simulink library "thc"  (R2021b)
settings: Solver=VariableStepAuto  StartTime=0.0  StopTime=10.0  RelTol=1e-3
undefined symbols (not defined in the file or in its folder): ATHC_APTCQA_X_C, ATHC_APTCQB_X_C, ATHC_dAy_X_C, ATHC_Qeq_X_kmh, ATHC_VbaseC_X_C, ATHC_VbaseC_Y_W, ATHC_VbaseD_X_C, ATHC_VbaseH_X_C, FALSE, KTHC_ACMaxMinT_sec, KTHC_aDeice_K, KTHC_AGSDefLv_K, KTHC_AGSLv1_K, KTHC_AGSLv2_K, KTHC_AGSLv3_K, KTHC_AGSLv4_K, KTHC_AGSLv5_K, KTHC_AirIntUpdateT_sec, KTHC_APTCOneZoneMax_W, KTHC_APTCQMaxC_W, KTHC_APTCQminC_W, KTHC_APTCQminD_W, KTHC_APTCQminRe1_W, KTHC_APTCQminRe_W, KTHC_APTCQoffT_cnt, KTHC_APTCQonT_cnt, KTHC_APTCRiLeMaxDff_W, KTHC_APTCRiLeMinDff_W, KTHC_BatInTempDef_C, KTHC_bDeice_K, KTHC_CompMaxDeice_rpm, KTHC_CompMinDeice_rpm, KTHC_CompSotxvOp_K, KTHC_CompSotxvOpLow_rpm, KTHC_CompSpdmax_rpm, KTHC_CompSpdmaxBC1_rpm, KTHC_CompSpdmaxBC_rpm, KTHC_CompSpdmid1_rpm, KTHC_CompSpdmid2_rpm, KTHC_CompSpdmid3_rpm, KTHC_CompSpdmid_rpm, KTHC_CompSpdmin_rpm, KTHC_DAPTCQ1_W, KTHC_DAPTCQ2_W, KTHC_DAPTCQ3_W, KTHC_DcChSetTemp_C, KTHC_DehumidityEN_flg, KTHC_DeiceCycTime_K, KTHC_DTambSat1_C, KTHC_DTambSat2_C, KTHC_DTambsat3_C, KTHC_DTambsat4_C, KTHC_DTambSat5_C, KTHC_DTambSat_C, KTHC_DTcabin10_C, KTHC_DTCabin11_C, KTHC_DTcabin12_C, KTHC_DTcabin1_C, KTHC_DTcabin2_C, KTHC_DTcabin3_C ... (+347)
libraries: simulink x80
(part 6 of 8)

== stateflow chart thc/THC/ThermalControl/AC/Chart ==
  state Sync [parallel]
    settings: executionOrder=1
    state WaitForIVI
    state Release
    state Press
      state Wait
      state Over10sec
        en:ACForceOFF=!ACForceOFF;
      (default) -> Wait
      Wait -> Over10sec : [after(100,tick)]
    (default) -> WaitForIVI : {CCU_SyncSts=EEP_CCUSyncSts;ACForceOFF=EEP_ACForceOFF;}
    WaitForIVI -> Sync.Release : [VINP_CANMsgValidIVI2_flg]
    Sync.Release -> Sync.Release [order 2] : [hasChanged(sigSetTempZon2Req_CMD)&&....
        | (sigSetTempZon2Req_CMD) != (sigSetTempZon1Req_CMD)]
        | {CCU_SyncSts=false;}
    Sync.Release -> Sync.Press [order 1] : [FCP_FrEvt_BtnSyncReq]
        | {CCU_SyncSts=!CCU_SyncSts;}
    Sync.Press -> Sync.Release [order 1] : [!FCP_FrEvt_BtnSyncReq]
    Sync.Press -> Sync.Press [order 2] : [hasChanged(sigSetTempZon2Req_CMD)&&....
        | (sigSetTempZon2Req_CMD) != (sigSetTempZon1Req_CMD)]
        | {CCU_SyncSts=false;}
  state Recycle [parallel]
    settings: executionOrder=13
    state Manual
      state Outter
        en:sigRecircSt=false;
        state ACOFF
          en:FD_RecyAuto_Cmd=0;
        state ACON
          en:FD_RecyAuto_Cmd=4;
        (default) -> (junction 1044)
        (junction 1044) -> ACOFF [order 1] : [!CCU_ACLampSts&&....
            | (CabinMode==11&&....
            | ACSubMode==1)]
        (junction 1044) -> ACON [order 2]
        ACON -> ACOFF : [!CCU_ACLampSts&&....
            | (CabinMode==11&&ACSubMode==1)]
        ACOFF -> ACON : [CCU_ACLampSts||....
            | (CabinMode!=11||ACSubMode!=1)]
      state Inner
        en:sigRecircSt=true;
        FD_RecyAuto_Cmd=0;
      (default) -> (junction 920)
      (junction 920) -> (junction 922) [order 1] : [EEP_sigRecircSt]
      (junction 920) -> Outter [order 2]
      (junction 922) -> Inner
      Inner -> Outter [order 2] : eDefogRecycle
      Outter -> Inner : eRecycleBtn
      Inner -> Outter [order 1] : eRecycleBtn
      (junction 839) -> Outter [order 1] : [sigRecircSt]
      (junction 839) -> Inner [order 2]
    state Auto
      state SetLowT
        en:sigRecircSt=false;FD_RecyAuto_Cmd=4;
      state Normal
        state AutoInner
          en:
          sigRecircSt=true;
          note: 2 min
          state Refresh
            en:
            FD_RecyAuto_Cmd=4;
          state Hold
            en:
            FD_RecyAuto_Cmd=0;
          (default) -> Hold
          Refresh -> Hold : [after(KTHC_RecyChange_min*600,tick)]
          Hold -> Refresh : [KTHC_RefreshEN_flg&&...
              | after(KTHC_RecyHold_min*600,tick)]
        note: 30 min
        state AutoOutter
          en:sigRecircSt=false;
          state Dehumidity
            en:FD_RecyAuto_Cmd=KTHC_RecyOutterD_enum;
          state Normal
            state LV5
              en:FD_RecyAuto_Cmd=4;
            state LV4
              en:FD_RecyAuto_Cmd=3;
            state LV3
              en:FD_RecyAuto_Cmd=2;
            state LV2
              en:FD_RecyAuto_Cmd=1;
            (junction 713) -> LV5 [order 1] : [Tamb>KTHC_T4Mmaxamb_C]
            (junction 713) -> (junction 719) [order 2]
            LV5 -> LV4 : [Tamb<KTHC_T5Mminamb_C]
            LV4 -> LV5 [order 1] : [Tamb>KTHC_T4Mmaxamb_C]
            (junction 719) -> LV4 [order 1] : [Tamb>KTHC_T3Mmaxamb_C]
            (junction 719) -> (junction 725) [order 2]
            LV4 -> LV3 [order 2] : [Tamb<KTHC_T4Mminamb_C]
            LV3 -> LV4 [order 1] : [Tamb>KTHC_T3Mmaxamb_C]
            (junction 725) -> LV3 [order 1] : [Tamb>KTHC_T2Mmaxamb_C]
            (junction 725) -> (junction 730) [order 2]
            LV3 -> LV2 [order 2] : [Tamb<KTHC_T3Mminamb_C]
            LV2 -> LV3 : [Tamb>KTHC_T2Mmaxamb_C]
            (junction 730) -> LV2
          (default) -> (junction 1030)
          (junction 1030) -> Dehumidity [order 1] : [CabinMode<7]
          (junction 1030) -> (junction 1034) [order 2]
          Dehumidity -> (junction 1034) : [CabinMode>=7]
          (junction 1034) -> (junction 713)
          Recycle.Auto.Normal.AutoOutter.Normal -> Dehumidity : [CabinMode<7]
        (default) -> (junction 752)
        (junction 752) -> AutoInner [commented out] : [CabinMode==3||....
            | CabinMode==6||....
            | (CabinMode==11&&....
            | ACSubMode==1)]
        (junction 752) -> (junction 754)
        AutoInner -> (junction 754) : [CabinMode!=3&&....
            | CabinMode!=6&&....
            | (CabinMode!=11||....
            | ACSubMode!=1)]
        (junction 754) -> AutoOutter
        AutoOutter -> AutoInner : [CabinMode==3||CabinMode==6||....
            | (CabinMode==11&&ACSubMode==1)]
      (default) -> (junction 1010)
      (junction 1010) -> (junction 1014) [order 1]
      (junction 1014) -> SetLowT : [CabinMode==3&&(ACSubMode==2||ACSubMode==6||ACSubMode==7)....
          | &&SetTempZon1St_CMD==170&&Tamb<KTHC_Trecymin_C]
      SetLowT -> Recycle.Auto.Normal : [CabinMode!=3||(ACSubMode!=2&&ACSubMode!=6&&ACSubMode!=7)||....
          | SetTempZon1St_CMD>170||Tamb>=KTHC_Trecymin_C]
      (junction 1010) -> Recycle.Auto.Normal [order 2]
      Recycle.Auto.Normal -> (junction 1014)
    (default) -> (junction 914)
    (junction 914) -> Recycle.Manual [order 1] : [EEP_ACModeMem!=2||!EEP_RecAutoFlg]
        | {RecAutoFlg=EEP_RecAutoFlg;}
    (junction 914) -> (junction 917) [order 2]
    Recycle.Auto -> (junction 839) [order 3] : eRecycleBtn
    Recycle.Auto -> Outter [order 2] : [!CCU_AutoLampSts&&!RecAutoFlg&&!sigRecircSt]
    Recycle.Auto -> Outter [order 1] : eDefogRecycle
    Recycle.Auto -> Inner [order 4] : [!CCU_AutoLampSts&&!RecAutoFlg]
    Recycle.Manual -> Recycle.Auto [order 2] : eACMaxRec
    Recycle.Manual -> Recycle.Auto [order 1] : [CCU_AutoLampSts&&RecAutoFlg]
    (junction 917) -> Recycle.Auto
  state RecycleSW [parallel]
    settings: executionOrder=14
    state Release
    state Press
      en:Recycle.eRecycleBtn;
      RecAutoFlg=false;
    (default) -> RecycleSW.Release
    RecycleSW.Release -> RecycleSW.Press : [sigRecircReq]
    RecycleSW.Press -> RecycleSW.Release : [!sigRecircReq]
  state PETMODE [parallel]
    settings: executionOrder=16
    state OFF
      en:PET=false;
    state ON
      en:PET=true;
    (default) -> PETMODE.OFF
    PETMODE.OFF -> PETMODE.ON : [(PwrSta>0&&PwrSta<=3&&(OFF_AC_MODE==1||OFF_AC_MODE==2||VINP_RemoteAutoReq_flg))||(ForceAuto&&PwrSta>3)]
    PETMODE.ON -> PETMODE.OFF : [(PwrSta==0||PwrSta>3||(OFF_AC_MODE!=1&&OFF_AC_MODE!=2&&!VINP_RemoteAutoReq_flg))&&(!ForceAuto||PwrSta<=3)]
  state ACBtn [parallel]
    settings: executionOrder=2
    state Initial
    state Release
    state Press
      en:AC.ACMode.eACBtn;
      WaterFill.eACBtn;
    (default) -> ACBtn.Initial
    ACBtn.Initial -> (junction 899) [order 2]
    (junction 899) -> ACBtn.Press
    ACBtn.Initial -> ACBtn.Release [order 1] : [EEP_ACModeMem!=1]
    ACBtn.Press -> ACBtn.Release : [!FCP_FrEvt_BtnACReq]
    ACBtn.Release -> ACBtn.Press : [FCP_FrEvt_BtnACReq]
  state ACAutoBtn [parallel]
    settings: executionOrder=3
    state Initial
    state Release
    state Press
      en:
      WaterFill.eACAutoBtn;
      RecAutoFlg=true;
    (default) -> ACAutoBtn.Initial
    ACAutoBtn.Initial -> (junction 904) [order 2] : {AC.ACMode.eACAutoBtn;}
    (junction 904) -> ACAutoBtn.Release
    ACAutoBtn.Initial -> ACAutoBtn.Release [order 1] : [EEP_ACModeMem!=2]
    ACAutoBtn.Release -> (junction 700) : [FCP_FrEvt_BtnAutoReq]
    (junction 700) -> ACAutoBtn.Press [order 1] : [CCU_AutoLampSts]{AC.ACMode.eAutoexit;}
    (junction 700) -> (junction 702) [order 2]
    (junction 702) -> ACAutoBtn.Press : {AC.ACMode.eACAutoBtn;}
    ACAutoBtn.Press -> ACAutoBtn.Release : [!FCP_FrEvt_BtnAutoReq]
  state ACMaxBtn [parallel]
    settings: executionOrder=4
    state Release
    state Press
      en:AC.ACMode.eACMaxBtn;
    (default) -> ACMaxBtn.Release
    ACMaxBtn.Release -> ACMaxBtn.Press : [FCP_FrEvt_BtnACMaxReq]
    ACMaxBtn.Press -> ACMaxBtn.Release : [!FCP_FrEvt_BtnACMaxReq]
  state FaceBtn [parallel]
    settings: executionOrder=5
    state Press
      en:AC.ACMode.eAutoexit;
    state Release
    (default) -> FaceBtn.Release : {Face=EEP_Face;}
    FaceBtn.Press -> FaceBtn.Release : [!sigFaceReq]
    FaceBtn.Release -> (junction 183) : [sigFaceReq]{fdefog=false;}
    (junction 183) -> FaceBtn.Press [order 1] : [Face&&!Foot&&!Frost]
    (junction 183) -> (junction 185) [order 2]
    (junction 185) -> FaceBtn.Press : {Face=!Face;}
  state FootBtn [parallel]
    settings: executionOrder=6
    state Release
    state Press
      en:AC.ACMode.eAutoexit;
    (default) -> FootBtn.Release : {Foot=EEP_Foot;}
    FootBtn.Press -> FootBtn.Release : [!sigFootReq]
    FootBtn.Release -> (junction 189) : [sigFootReq]{fdefog=false;}
    (junction 189) -> FootBtn.Press [order 1] : [!Face&&Foot&&!Frost]
    (junction 189) -> (junction 197) [order 2]
    (junction 197) -> FootBtn.Press : {Foot=!Foot;}
  state Frost [parallel]
    settings: executionOrder=7
    state Press
      en:AC.ACMode.eAutoexit;
      ACModeMem=1;
    state Release
    (default) -> Frost.Release : {Frost=EEP_Frost;FaceM=EEP_FaceM;FootM=EEP_FootM;fdefog=EEP_fdefog;}
    Frost.Press -> Frost.Release : [!sigFrostReq]
    Frost.Release -> (junction 206) : [sigFrostReq]
    (junction 206) -> Frost.Press [order 1] : [!Frost]{Frost=true;FaceM=Face;FootM=Foot;....
        | Face=false;Foot=false;fdefog=true;Recycle.eDefogRecycle;RecAutoFlg=false;}
    (junction 206) -> (junction 200) [order 2]
    (junction 200) -> Frost.Press [order 1] : [!Face&&!Foot]{Frost=false;Face=FaceM;Foot=FootM;fdefog=false;}
    (junction 200) -> (junction 769) [order 2]
    (junction 769) -> Frost.Press : {Frost=false;fdefog=false;}
  state AC [parallel]
    settings: executionOrder=15
    state ACMode
      state ON
        state Max
          en:
          CCU_ACLampSts=true;
          CCU_AutoLampSts=false;
          CCU_ACMaxLampSts=true;
          sigAirIntenZon1St=9;
          CCU_SyncSts=true;
          Recycle.eACMaxRec;
          RecAutoFlg=true;
          state WaitMinT
          state WaitFinish
          (default) -> WaitMinT
          WaitMinT -> WaitFinish : [after(KTHC_ACMaxMinT_sec*10,tick)]
        state Manual
          en:
          CCU_ACLampSts=true;CCU_AutoLampSts=false;
          CCU_ACMaxLampSts=false;ACModeMem=1;
          RecAutoFlg=false;
          ACModeMem = 1;
          state Normal
            en:
            sigAirIntenZon1St=AirIntenZone1M;
            du:
            sigAirIntenZon1St=AirIntenZone1M;
          state DeFog
            en:
            sigAirIntenZon1St=9;
            ex:
            fdefog=false;
          (default) -> (junction 779)
          (junction 779) -> DeFog [order 2]
          (junction 779) -> AC.ACMode.ON.Manual.Normal [order 1] : [!fdefog]
          DeFog -> AC.ACMode.ON.Manual.Normal : [!fdefog]
          AC.ACMode.ON.Manual.Normal -> DeFog : [fdefog]
        state Auto
          en:
          CCU_ACLampSts=true;
          CCU_AutoLampSts=true;
          CCU_ACMaxLampSts=false;
          ACModeMem=2;
        WaitFinish -> (junction 851) : [MaxFinish||....
            | !CCU_SyncSts]
        Max -> AC.ACMode.ON.Manual [order 2] : eACMaxexit
        AC.ACMode.ON.Manual -> Max : eACMaxBtn
        Max -> (junction 850) [order 1] : eACMaxBtn
        AC.ACMode.ON.Auto -> Max [order 1] : eACMaxBtn
        (junction 850) -> (junction 851)
        (junction 851) -> (junction 49)
        (junction 49) -> AC.ACMode.ON.Manual [order 2]
        (junction 49) -> AC.ACMode.ON.Auto [order 1] : [ACModeMem==2]
        AC.ACMode.ON.Auto -> AC.ACMode.ON.Manual [order 2] : eAutoexit
        AC.ACMode.ON -> AC.ACMode.ON.Auto [order 1] : eACAutoBtn
        (default) -> (junction 943)
        (junction 943) -> AC.ACMode.ON.Manual [order 2]
        (junction 943) -> AC.ACMode.ON.Auto [order 1] : [ACModeMem == 2]
      state OFF
        en:
        CCU_ACLampSts=false;
        CCU_AutoLampSts=false;
        CCU_ACMaxLampSts=false;
        ACModeMem=0;
        sigAirIntenZon1St=AirIntenZone1M;
        du:
        sigAirIntenZon1St=AirIntenZone1M;
      (default) -> AC.ACMode.OFF
      AC.ACMode.OFF -> (junction 669) [order 4] : eACMaxBtn{ACModeMem=1;}
      (junction 669) -> Max [order 1] : [AirIntenZone1M!=1]
      (junction 669) -> (junction 671) [order 2]
      (junction 671) -> Max : {AirIntenZone1M=2;}
      AC.ACMode.ON -> AC.ACMode.OFF [order 1] : eACBtn
      AC.ACMode.OFF -> (junction 832) [order 2] : eACBtn
      (junction 832) -> (junction 833)
      AC.ACMode.OFF -> (junction 833) [order 1] : [fdefog]
      (junction 833) -> (junction 674)
      (junction 674) -> AC.ACMode.ON.Manual [order 1] : [AirIntenZone1M!=1]
      (junction 674) -> (junction 677) [order 2]
      (junction 677) -> AC.ACMode.ON.Manual : {AirIntenZone1M=2;}
      AC.ACMode.ON -> AC.ACMode.OFF [order 2] : [sigAirIntenZon1Req==1]
      (junction 683) -> AC.ACMode.ON.Auto [order 1] : [AirIntenZone1M!=1]
      AC.ACMode.OFF -> (junction 683) [order 3] : eACAutoBtn
      (junction 683) -> (junction 680) [order 2]
      (junction 680) -> AC.ACMode.ON.Auto : {AirIntenZone1M=2;}
      (junction 948) -> AC.ACMode.OFF [order 1] : [ACModeMem == 0]
      (junction 948) -> AC.ACMode.ON [order 2]
      (junction 947) -> (junction 948)
    state PET
      en:
      CCU_ACLampSts=true;
      CCU_AutoLampSts=true;
      CCU_ACMaxLampSts=false;
    (default) -> ACMode
    ACMode -> PET : [PET]
    PET -> (junction 947) : [!PET]
  state AutoWindDir [parallel]
    settings: executionOrder=12
    state Manmual
    state Standby
    (default) -> (junction 560)
    (junction 560) -> Manmual [order 1] : [!CCU_AutoLampSts]
    (junction 560) -> (junction 871) [order 2]
    Standby -> (junction 871) [order 3] : [hasChanged(VTHC_FootCold_flg)]
    (junction 871) -> (junction 578)
    Manmual -> (junction 578) : [CCU_AutoLampSts]
    Standby -> (junction 578) [order 1] : [after(KTHC_WindDirUpdateT_min*600,tick)||hasChanged(SetTempZon1St_CMD)]
    (junction 578) -> (junction 562)
    (junction 562) -> (junction 568) [order 1] : [Tamb<20]
    (junction 568) -> Standby [order 1] : [sigSetTempZon1St<Tincar||VTHC_FootCold_flg]....
        | {Face=KTHC_WDZ2Face_flg;Foot=KTHC_WDZ2Foot_flg;Frost=KTHC_WDZ2Frost_flg;}
    (junction 562) -> (junction 573) [order 2]
    (junction 568) -> (junction 570) [order 2]
    (junction 570) -> Standby : {Face=KTHC_WDZ1Face_flg;Foot=KTHC_WDZ1Foot_flg;Frost=KTHC_WDZ1Frost_flg;}
    (junction 575) -> Standby [order 1] : [Tincar-Tamb>KTHC_Tmidlevel_C]....
        | {Face=KTHC_WDZ5Face_flg;Foot=KTHC_WDZ5Foot_flg;Frost=KTHC_WDZ5Frost_flg;}
    (junction 573) -> (junction 575) [order 1] : [Tamb<25]
    (junction 573) -> (junction 581) [order 2]
    (junction 575) -> (junction 605) [order 2]
    (junction 605) -> Standby [order 1] : [sigSetTempZon1St<Tincar||VTHC_FootCold_flg]....
        | {Face=KTHC_WDZ3Face_flg;Foot=KTHC_WDZ3Foot_flg;Frost=KTHC_WDZ3Frost_flg;}
    (junction 605) -> (junction 608) [order 2]
    (junction 608) -> Standby : {Face=KTHC_WDZ4Face_flg;Foot=KTHC_WDZ4Foot_flg;Frost=KTHC_WDZ4Frost_flg;}
    (junction 624) -> Standby [order 1] : [sigSetTempZon1St<Tincar]....
        | {Face=KTHC_WDZ9Face_flg;Foot=KTHC_WDZ9Foot_flg;Frost=KTHC_WDZ9Frost_flg;}
    (junction 581) -> (junction 624) [order 1] : [Tincar-Tamb>KTHC_Thilevel2_C]
    (junction 581) -> (junction 583) [order 2]
    (junction 624) -> (junction 625) [order 2]
    (junction 625) -> Standby : {Face=KTHC_WDZ8Face_flg;Foot=KTHC_WDZ8Foot_flg;Frost=KTHC_WDZ8Frost_flg;}
    (junction 1051) -> (junction 625) [order 2]
    (junction 583) -> (junction 1051) [order 1] : [Tincar-Tamb>KTHC_Thilevel1_C]
    (junction 1051) -> Standby [order 1] : [sigSetTempZon1St<Tincar]....
        | {Face=KTHC_WDZ10Face_flg;Foot=KTHC_WDZ10Foot_flg;Frost=KTHC_WDZ10Frost_flg;}
    (junction 583) -> (junction 586) [order 2]
    (junction 586) -> Standby [order 1] : [sigSetTempZon1St>=Tincar]....
        | {Face=KTHC_WDZ7Face_flg;Foot=KTHC_WDZ7Foot_flg;Frost=KTHC_WDZ7Frost_flg;}
    (junction 586) -> (junction 589) [order 2]
    (junction 589) -> Standby : {Face=KTHC_WDZ6Face_flg;Foot=KTHC_WDZ6Foot_flg;Frost=KTHC_WDZ6Frost_flg;}
    Standby -> Manmual [order 2] : [!CCU_AutoLampSts]
  state WindDir [parallel]
    settings: executionOrder=8
    state Face
      en:sigWindDirZon1St=0;
    state Bilevel
      en:sigWindDirZon1St=1;
    state Foot
      en:sigWindDirZon1St=2;
    state FootandScreen
      en:sigWindDirZon1St=3;
    state Defog
      en:sigWindDirZon1St=4;
    state FaceandScreen
      en:sigWindDirZon1St=5;
    state AllOpen
      en:sigWindDirZon1St=6;
    state AllClose
      en:sigWindDirZon1St=7;
    (default) -> (junction 457)
    WindDir -> (junction 457) : [hasChanged(Face)||....
        | hasChanged(Foot)||....
        | hasChanged(Frost)]
    (junction 457) -> Face [order 1] : [Face&&!Foot&&!Frost]
    (junction 457) -> (junction 464) [order 2]
    (junction 464) -> Bilevel [order 1] : [Face&&Foot&&!Frost]
    (junction 464) -> (junction 467) [order 2]
    (junction 467) -> Foot [order 1] : [!Face&&Foot&&!Frost]
    (junction 467) -> (junction 472) [order 2]
    (junction 472) -> FootandScreen [order 1] : [!Face&&Foot&&Frost]
    (junction 472) -> (junction 476) [order 2]
    (junction 476) -> Defog [order 1] : [!Face&&!Foot&&Frost]
    (junction 476) -> (junction 480) [order 2]
    (junction 480) -> FaceandScreen [order 1] : [Face&&!Foot&&Frost]
    (junction 480) -> (junction 484) [order 2]
    (junction 484) -> AllOpen [order 1] : [Face&&Foot&&Frost]
    (junction 484) -> AllClose [order 2]
  state Manual [parallel]
    settings: executionOrder=10
    state Updated
      en:AC.ACMode.eAutoexit;
      CCU_AutoLampSts=false;
    state Auto
      state WaitForUpdate
      (default) -> (junction 953) : {FAutoFirst=true;}
      WaitForUpdate -> (junction 953) [order 2] : [after(2,tick)&&FAutoFirst]{FAutoFirst=false;}
      (junction 953) -> (junction 954)
      WaitForUpdate -> (junction 954) [order 3] : [FD_Blower_Cmd>AirIntHB||FD_Blower_Cmd<AirIntLB]
      (junction 954) -> (junction 955)
      WaitForUpdate -> (junction 955) [order 1] : [after(KTHC_AirIntUpdateT_sec*10,tick)]
      (junction 955) -> (junction 956)
      (junction 956) -> WaitForUpdate [order 1] : [FD_Blower_Cmd>=94]{sigAirIntenZon1St=9;AirIntLB=87.5;AirIntHB=100;}
      (junction 956) -> (junction 957) [order 2]
      (junction 957) -> WaitForUpdate [order 1] : [FD_Blower_Cmd>=82]{sigAirIntenZon1St=8;AirIntLB=75;AirIntHB=100;}
      (junction 957) -> (junction 958) [order 2]
      (junction 958) -> WaitForUpdate [order 1] : [FD_Blower_Cmd>=69]{sigAirIntenZon1St=7;AirIntLB=62.5;AirIntHB=87.5;}
      (junction 958) -> (junction 959) [order 2]
      (junction 959) -> WaitForUpdate [order 1] : [FD_Blower_Cmd>=56]{sigAirIntenZon1St=6;AirIntLB=50;AirIntHB=75;}
      (junction 959) -> (junction 960) [order 2]
      (junction 960) -> WaitForUpdate [order 1] : [FD_Blower_Cmd>=44]{sigAirIntenZon1St=5;AirIntLB=37.5;AirIntHB=62.5;}
      (junction 960) -> (junction 961) [order 2]
      (junction 961) -> WaitForUpdate [order 1] : [FD_Blower_Cmd>=32]{sigAirIntenZon1St=4;AirIntLB=25;AirIntHB=50;}
      (junction 961) -> (junction 962) [order 2]
      (junction 962) -> WaitForUpdate [order 1] : [FD_Blower_Cmd>=19]{sigAirIntenZon1St=3;AirIntLB=12.5;AirIntHB=37.5;}
      (junction 962) -> (junction 963) [order 2]
      (junction 963) -> WaitForUpdate : {sigAirIntenZon1St=2;;AirIntLB=0;AirIntHB=25;}
    (default) -> (junction 117) : {AirIntenZone1M=EEP_AirIntenZone1M;}
    (junction 117) -> Updated [order 2]
    (junction 117) -> Manual.Auto [order 1] : [CCU_AutoLampSts]
    Updated -> Manual.Auto : [CCU_AutoLampSts]
    Manual.Auto -> Updated : [!CCU_AutoLampSts]
    (junction 817) -> Updated [order 1] : [CCU_ACMaxLampSts]....
        | {AC.ACMode.eACMaxexit;}
    Manual -> (junction 817) : [hasChanged(sigAirIntenZon1Req)&&....
        | sigAirIntenZon1Req>0&&sigAirIntenZon1Req<10]....
        | {AirIntenZone1M=sigAirIntenZon1Req;fdefog=false;}
    (junction 817) -> (junction 819) [order 2]
    (junction 819) -> Updated
  state WaterFill [parallel]
    settings: executionOrder=9
    state Count1
    state OFF
      en:WaterFillReq=0;
      WFCnt=0;
    state Count
      en:WFCnt=WFCnt+1;
    state WaterFill2
      en:WaterFillReq=2;
    state WaterFill1
      en:WaterFillReq=1;
    (default) -> WaterFill.OFF
    WaterFill.OFF -> Count1 [order 2] : [FCP_FrEvt_BtnACReq]
    Count1 -> WaterFill.OFF [order 1] : [!FCP_FrEvt_BtnACReq]
    WaterFill.OFF -> Count [order 1] : eACAutoBtn....
        | [SetTempZon1St_CMD == 220 &&...
        |  SetTempZon2St_CMD == 310]
    Count -> WaterFill.OFF [order 3] : [SetTempZon1St_CMD != 220 ||...
        |  SetTempZon2St_CMD !=310 ||...
        | after(20,tick)]
    WaterFill1 -> WaterFill.OFF [order 1] : eACBtn
    (junction 1005) -> WaterFill.OFF : eACAutoBtn
    (junction 1002) -> WaterFill.OFF [order 1] : [after(36000,tick)||....
        | PwrSta==0||....
        | PwrSta==5]
    Count1 -> WaterFill2 [order 2] : [after(50,tick)]
    Count -> Count [order 2] : eACAutoBtn
    Count -> WaterFill1 [order 1] : [WFCnt>=3]
    (junction 1002) -> (junction 1005) [order 2]
    WaterFill2 -> (junction 1002)
    WaterFill1 -> (junction 1002) [order 2]
  state TFootUpdate [parallel]
    settings: executionOrder=11
    state Low
      en:
      VTHC_FootCold_flg=true;
    state High
      en:
      VTHC_FootCold_flg=false;
    (default) -> (junction 864)
    (junction 864) -> Low [order 1] : [T_Foot_min<KTHC_FootColdT_C]
    (junction 864) -> High [order 2]
    High -> Low : [T_Foot_min<KTHC_FootColdT_C]
    Low -> High : [T_Foot_min>KTHC_FootColdT_C+KTHC_FootColdTdelta_C]
  data: FCP_FrEvt_BtnACMaxReq input; FCP_FrEvt_BtnACReq input; FCP_FrEvt_BtnAutoReq input; FCP_FrEvt_BtnSyncReq input; FD_Blower_Cmd input; Tamb input; Tincar input; sigAirIntenZon1Req input; sigRecircReq input; CCU_ACLampSts output boolean; CCU_ACMaxLampSts output boolean; CCU_SyncSts output; sigAirIntenZon1St output; sigWindDirZon1St output; CCU_AutoLampSts output boolean; sigRecircSt output =0; sigFaceReq input; sigFootReq input; sigFrostReq input; sigSetTempZon1St input; SetTempZon1St_CMD input; sigSetTempZon2St input; SetTempZon2St_CMD input; PwrSta input; sigSetTempZon1Req input; sigSetTempZon2Req_CMD input; sigSetTempZon1Req_CMD input; sigSetTempZon2Req input; WaterFillReq output uint8; WFCnt local uint8; Frost output boolean; ACForceOFF output; KTHC_WindDirUpdateT_min input; KTHC_AirIntUpdateT_sec input; OFF_AC_MODE input; PET output boolean; FD_RecyAuto_Cmd output; KTHC_T2Mmaxamb_C input; KTHC_T3Mmaxamb_C input; KTHC_T4Mmaxamb_C input; KTHC_T3Mminamb_C input; KTHC_T4Mminamb_C input; KTHC_T5Mminamb_C input; KTHC_RecyHold_min input; KTHC_RecyChange_min input; KTHC_Tmidlevel_C input; KTHC_Thilevel1_C input; KTHC_Thilevel2_C input; CabinMode input; KTHC_WDZ1Face_flg input boolean; KTHC_WDZ1Foot_flg input boolean; KTHC_WDZ1Frost_flg input boolean; KTHC_WDZ2Face_flg input boolean; KTHC_WDZ2Foot_flg input boolean; KTHC_WDZ2Frost_flg input boolean; KTHC_WDZ3Face_flg input boolean; KTHC_WDZ3Foot_flg input boolean; KTHC_WDZ3Frost_flg input boolean; KTHC_WDZ4Face_flg input boolean; KTHC_WDZ4Foot_flg input boolean; KTHC_WDZ4Frost_flg input boolean; KTHC_WDZ5Face_flg input boolean; KTHC_WDZ5Foot_flg input boolean; KTHC_WDZ5Frost_flg input boolean; KTHC_WDZ6Face_flg input boolean; KTHC_WDZ6Foot_flg input boolean; KTHC_WDZ6Frost_flg input boolean; KTHC_WDZ7Face_flg input boolean; KTHC_WDZ7Foot_flg input boolean; KTHC_WDZ7Frost_flg input boolean; KTHC_WDZ8Face_flg input boolean; KTHC_WDZ8Foot_flg input boolean; KTHC_WDZ8Frost_flg input boolean; KTHC_WDZ9Face_flg input boolean; KTHC_WDZ9Foot_flg input boolean; KTHC_WDZ9Frost_flg input boolean; KTHC_WDZ10Face_flg input; KTHC_WDZ10Foot_flg input; KTHC_WDZ10Frost_flg input; ForceAuto input; KTHC_RefreshEN_flg input boolean; MaxFinish input; T_Foot_min input; KTHC_FootColdT_C input; KTHC_FootColdTdelta_C input; VTHC_FootCold_flg local boolean; KTHC_ACMaxMinT_sec input; FAutoFirst local boolean; ACModeMem output; EEP_ACModeMem input; EEP_Face input; EEP_Foot input; EEP_Frost input; EEP_FaceM input; EEP_FootM input; FaceM output boolean; FootM output boolean; Face output boolean; Foot output boolean; EEP_CCUSyncSts input; EEP_ACForceOFF input; EEP_sigRecircSt input; EEP_RecAutoFlg input; EEP_AirIntenZone1M input; EEP_fdefog input; fdefog output boolean; RecAutoFlg output boolean; AirIntenZone1M output; VINP_CANMsgValidIVI2_flg input; VINP_RemoteAutoReq_flg input; AirIntHB local double; AirIntLB local double; KTHC_Trecymin_C input; ACSubMode input; KTHC_RecyOutterD_enum input
  events: eRecycleBtn local FUNCTION_CALL_EVENT; eDefogRecycle local FUNCTION_CALL_EVENT; eACMaxRec local FUNCTION_CALL_EVENT; eACBtn local FUNCTION_CALL_EVENT; eACMaxBtn local FUNCTION_CALL_EVENT; eACAutoBtn local FUNCTION_CALL_EVENT; eAutoexit local FUNCTION_CALL_EVENT; eACMaxexit local FUNCTION_CALL_EVENT; eACAutoBtn local FUNCTION_CALL_EVENT; eACBtn local FUNCTION_CALL_EVENT

== stateflow chart thc/THC/ThermalControl/THCM_Conctrl/Chart2 ==
  state FactorSolar1
    en:FactorSolar=0.88;Blowersolar=1000;
    state Low
    state Mid
    (default) -> FactorSolar1.Mid
    FactorSolar1.Mid -> FactorSolar1.Low : [Solar<950]
    FactorSolar1.Low -> FactorSolar1.Mid [order 1] : [Solar>=950]
  state FactorSolar2
    en:FactorSolar=0.90;Blowersolar=860;
    state Low
    state Mid
    state High
    (default) -> FactorSolar2.Mid
    FactorSolar2.Mid -> FactorSolar2.High [order 2] : [Solar>1000]
    FactorSolar2.Mid -> FactorSolar2.Low [order 1] : [Solar<800]
    FactorSolar2.Low -> FactorSolar2.Mid [order 1] : [Solar>=800]
    FactorSolar2.High -> FactorSolar2.Mid [order 2] : [Solar<=1000]
  state FactorSolar3
    en:FactorSolar=0.92;Blowersolar=715;
    state Low
    state Mid
    state High
    (default) -> FactorSolar3.Mid
    FactorSolar3.Mid -> FactorSolar3.High [order 2] : [Solar>850]
    FactorSolar3.Mid -> FactorSolar3.Low [order 1] : [Solar<650]
    FactorSolar3.Low -> FactorSolar3.Mid [order 1] : [Solar>=650]
    FactorSolar3.High -> FactorSolar3.Mid [order 1] : [Solar<=850]
  state FactorSolar4
    en:FactorSolar=0.94;Blowersolar=570;
    state Low
    state Mid
    state High
    (default) -> FactorSolar4.Mid
    FactorSolar4.Mid -> FactorSolar4.High [order 2] : [Solar>700]
    FactorSolar4.Mid -> FactorSolar4.Low [order 1] : [Solar<500]
    FactorSolar4.Low -> FactorSolar4.Mid [order 1] : [Solar>=500]
    FactorSolar4.High -> FactorSolar4.Mid [order 1] : [Solar<=700]
  state FactorSolar5
    en:FactorSolar=0.96;Blowersolar=430;
    state Low
    state Mid
    state High
    (default) -> FactorSolar5.Mid
    FactorSolar5.Mid -> FactorSolar5.High [order 2] : [Solar>550]
    FactorSolar5.Mid -> FactorSolar5.Low [order 1] : [Solar<350]
    FactorSolar5.Low -> FactorSolar5.Mid [order 1] : [Solar>=350]
    FactorSolar5.High -> FactorSolar5.Mid [order 1] : [Solar<=550]
  state FactorSolar6
    en:FactorSolar=0.98;Blowersolar=285;
    state Low
    state Mid
    state High
    (default) -> FactorSolar6.Mid
    FactorSolar6.Mid -> FactorSolar6.High [order 2] : [Solar>400]
    FactorSolar6.Mid -> FactorSolar6.Low [order 1] : [Solar<200]
    FactorSolar6.Low -> FactorSolar6.Mid : [Solar>=200]
    FactorSolar6.High -> FactorSolar6.Mid [order 1] : [Solar<=400]
  state FactorSolar7
    en:FactorSolar=1;Blowersolar=100;
    state Mid
    state High
    (default) -> FactorSolar7.Mid
    FactorSolar7.Mid -> FactorSolar7.High : [Solar>250]
    FactorSolar7.High -> FactorSolar7.Mid [order 1] : [Solar<=250]
  (default) -> (junction 9)
  (junction 9) -> FactorSolar1 [order 1] : [Solar>950]
  (junction 9) -> (junction 11) [order 2]
  FactorSolar1.Low -> FactorSolar2 [order 2] : [after(KTHC_SolarDebounceT_sec*10,tick)]
  FactorSolar2.High -> FactorSolar1 [order 1] : [after(KTHC_SolarDebounceT_sec*10,tick)]
  (junction 11) -> FactorSolar2 [order 1] : [Solar>800]
  (junction 11) -> (junction 14) [order 2]
  FactorSolar2.Low -> FactorSolar3 [order 2] : [after(KTHC_SolarDebounceT_sec*10,tick)]
  FactorSolar3.High -> FactorSolar2 [order 2] : [after(KTHC_SolarDebounceT_sec*10,tick)]
  (junction 14) -> FactorSolar3 [order 1] : [Solar>650]
  (junction 14) -> (junction 17) [order 2]
  FactorSolar3.Low -> FactorSolar4.Low [order 2] : [after(KTHC_SolarDebounceT_sec*10,tick)]
  FactorSolar4.High -> FactorSolar3 [order 2] : [after(KTHC_SolarDebounceT_sec*10,tick)]
  (junction 17) -> FactorSolar4 [order 1] : [Solar>500]
  (junction 17) -> (junction 20) [order 2]
  FactorSolar4.Low -> FactorSolar5.Low [order 2] : [after(KTHC_SolarDebounceT_sec*10,tick)]
  FactorSolar5.High -> FactorSolar4 [order 2] : [after(KTHC_SolarDebounceT_sec*10,tick)]
  (junction 20) -> FactorSolar5 [order 1] : [Solar>350]
  (junction 20) -> (junction 23) [order 2]
  FactorSolar5.Low -> FactorSolar6.Low [order 2] : [after(KTHC_SolarDebounceT_sec*10,tick)]
  FactorSolar6.High -> FactorSolar5 [order 2] : [after(KTHC_SolarDebounceT_sec*10,tick)]
  (junction 23) -> FactorSolar6 [order 1] : [Solar>200]
  (junction 23) -> (junction 26) [order 2]
  FactorSolar7.High -> FactorSolar6 [order 2] : [after(KTHC_SolarDebounceT_sec*10,tick)]
  (junction 26) -> FactorSolar7
  data: Solar input; FactorSolar output single; KTHC_SolarDebounceT_sec input; Blowersolar output

== stateflow chart thc/THC/ThermalControl/THCM_Conctrl/BlowerCtrl/SlowIncrease ==
  state OFF
    en:Bout=0;
  state ON
    state Increase
      en:Bout=KTHC_VBstep_K;
      du:Bout=Bout+KTHC_VBstep_K;
    state Operating
      en:Bout=Bin;
      du:Bout=Bin;
    Increase -> Operating : [Bin<Bout+KTHC_VBstep_K]
  (default) -> OFF
  OFF -> Increase : [Bin>0]
  ON -> OFF : [Bin<=0]
  data: Bin input; Bout output; KTHC_VBstep_K input

== stateflow chart thc/THC/ThermalControl/THCM_Conctrl/Chart ==
  state CabinModeDet [parallel]
    settings: executionOrder=1
    state CabinMode4or5
    state Heating
    state Else
    (default) -> (junction 50)
    (junction 50) -> CabinMode4or5 [order 1] : [CabinMode==4||CabinMode==5]
    (junction 50) -> (junction 54) [order 2]
    CabinMode4or5 -> Heating [order 1] : [CabinMode==8||CabinMode==9]
        | {Balance=true;}
    (junction 65) -> CabinMode4or5 : [CabinMode==4||....
        | CabinMode==5]
    CabinMode4or5 -> Else [order 2] : [CabinMode!=4&&....
        | CabinMode!=5]
    Heating -> (junction 65) [order 1]
    (junction 54) -> Heating [order 1] : [CabinMode==8||CabinMode==9]
    (junction 54) -> Else [order 2]
    Else -> (junction 65) [order 2]
    Else -> Heating [order 1] : [CabinMode==8||CabinMode==9]
    Heating -> Else [order 2] : [CabinMode!=8&&....
        | CabinMode!=9]
  state HighPBalance [parallel]
    settings: executionOrder=2
    state DeCrease
      en:CompOut=CompOut-Step;
      du:CompOut=CompOut-Step;
    state Finish
      en:CompOut=CompIn;
      SOTXVout=SOTXV;
      du:CompOut=CompIn;
      SOTXVout=SOTXV;
    (default) -> (junction 9)
    HighPBalance -> (junction 9) : [Balance]{Balance=false;}
    (junction 9) -> DeCrease [order 1] : [CompOut>KTHC_CompSotxvOpLow_rpm&&....
        | PT_High_P>KTHC_SotxvProHi_kPa]....
        | {Step=(CompOut-KTHC_CompSotxvOpLow_rpm)/KTHC_CompSotxvOp_K;}
    (junction 9) -> (junction 14) [order 2]
    DeCrease -> Finish : [CompOut<KTHC_CompSotxvOpLow_rpm&&....
        | PT_High_P<KTHC_SotxvProLo_kPa]
    (junction 14) -> Finish
  data: CabinMode input; CompIn input; Step local double; CompOut output =0; SOTXVout output boolean =false; KTHC_CompSotxvOpLow_rpm input; KTHC_CompSotxvOp_K input; KTHC_SotxvProHi_kPa input; KTHC_SotxvProLo_kPa input; PT_High_P input; Balance local boolean; SOTXV input

== stateflow chart thc/THC/ThermalControl/THCM_Conctrl/BlowerCtrl/Enabled Subsystem1/Chart2 ==
  state Voffset [parallel]
    settings: executionOrder=2
    state ACOFF
      state POWERon
        en:Voffset=Vmanual;
        du:Voffset=Vmanual;
      state OFF
        en:Voffset=0;
      (default) -> (junction 8)
      (junction 8) -> POWERon [order 2]
      (junction 8) -> OFF [order 1] : [CabinMode==0||....
          | PwrSta<=3]
      OFF -> POWERon : [CabinMode~=0&&PwrSta>3]
      POWERon -> OFF : [CabinMode==0||....
          | PwrSta<=3]
    state ACON
      state Defrst
        state Manual
          en:Voffset=Vmanual;
          du:Voffset=Vmanual;
        state Auto
          en:Voffset=KTHC_VBlowerdfog_K;
        (default) -> (junction 56)
        (junction 56) -> Voffset.ACON.Defrst.Auto [order 1] : [ACAuto]
        (junction 56) -> Voffset.ACON.Defrst.Manual [order 2]
        Voffset.ACON.Defrst.Manual -> Voffset.ACON.Defrst.Auto : [ACAuto]
        Voffset.ACON.Defrst.Auto -> Voffset.ACON.Defrst.Manual : [!ACAuto]
      state DefrstOFF
        state Auto
          state DontCorrect1
            en:Voffset=KTHC_VBlowerMin_K;
          state DontCorrect2
            en:Voffset=KTHC_VBlowerMid_K;
          state DontCorrect3
            en:Voffset=KTHC_VBlowerSetLow_K;
          state Vbase1
            en:Voffset=KTHC_VBlowerDcCh_K;
          state Vbase
            en:Voffset=Vbase;
            du:Voffset=Vbase;
          (default) -> (junction 104)
          Voffset.ACON.DefrstOFF.Auto -> (junction 104) [order 1] : [hasChanged(CabinMode)||....
              | hasChanged(ACSubMode)]
          (junction 104) -> DontCorrect1 [order 1] : [CabinMode==3&&ACSubMode==4]
          (junction 104) -> (junction 121) [order 2]
          (junction 121) -> DontCorrect2 [order 1] : [(CabinMode==3&&ACSubMode==5)||CabinMode==7]
          (junction 121) -> (junction 105) [order 2]
          (junction 105) -> DontCorrect3 [order 1] : [CabinMode==3&&....
              | (ACSubMode==6||ACSubMode==7||ACSubMode==0)]
          (junction 105) -> (junction 304) [order 2]
          (junction 304) -> Vbase1 [order 1] : [CabinMode==11]
          (junction 304) -> (junction 293) [order 2]
          (junction 293) -> Voffset.ACON.DefrstOFF.Auto.Vbase
        state Manual
          state DontCorrect
            en:Voffset=Vmanual;
            du:Voffset=Vmanual;
          state Vbase
            en:Voffset=Vbase;
            du:Voffset=Vbase;
          (default) -> (junction 83)
          Voffset.ACON.DefrstOFF.Manual -> (junction 83) [order 1] : [hasChanged(CabinMode)||....
              | hasChanged(ACSubMode)]
          (junction 83) -> DontCorrect [order 1] : [(CabinMode==3&&ACSubMode>=4)||CabinMode==7]
          (junction 83) -> (junction 91) [order 2]
          (junction 91) -> Voffset.ACON.DefrstOFF.Manual.Vbase
        (default) -> (junction 76)
        (junction 76) -> Voffset.ACON.DefrstOFF.Manual [order 2]
        (junction 76) -> Voffset.ACON.DefrstOFF.Auto [order 1] : [ACAuto]
        Voffset.ACON.DefrstOFF.Manual -> Voffset.ACON.DefrstOFF.Auto [order 1] : [ACAuto]
        Voffset.ACON.DefrstOFF.Auto -> Voffset.ACON.DefrstOFF.Manual [order 1] : [!ACAuto]
      (default) -> (junction 58)
      (junction 58) -> Defrst [order 1] : [DfrstReq]
      (junction 58) -> DefrstOFF [order 2]
      DefrstOFF -> Defrst : [DfrstReq]
      Defrst -> DefrstOFF : [!DfrstReq]
    (default) -> ACOFF
    ACOFF -> ACON : [CabinMode>2&&....
        | (CabinMode!=10||....
        | ACSubMode!=1)]
    ACON -> ACOFF : [CabinMode<=2||....
        | (CabinMode==10&&....
        | ACSubMode==1)]
  state VBase [parallel]
    settings: executionOrder=1
    state Cooling
      en:Vbase=VbaseC;
      du:Vbase=VbaseC;
    state Dehumidity
      en:Vbase=VbaseD;
      du:Vbase=VbaseD;
    state Heating
      en:Vbase=VbaseH;
      du:Vbase=VbaseH;
    state Vmanual
      en:Vbase=Vmanual;
      du:Vbase=Vmanual;
    (default) -> (junction 250)
    (junction 254) -> Cooling [order 1] : [CabinMode==3||....
        | (CabinMode==6&&ACSubMode==2)]
    VBase -> (junction 250) : [hasChanged(CabinMode)||....
        | hasChanged(ACAuto)]
    (junction 250) -> (junction 254) [order 1] : [ACAuto]
    (junction 250) -> Vmanual [order 2]
    (junction 254) -> (junction 258) [order 2]
    (junction 258) -> Dehumidity [order 1] : [CabinMode>3&&CabinMode<8]
    (junction 258) -> (junction 263) [order 2]
    (junction 263) -> Heating [order 1] : [CabinMode>=8]
    (junction 263) -> Vmanual [order 2]
  data: ACAuto input; ACSubMode input; CabinMode input; DfrstReq input; VbaseC input; VbaseD input; VbaseH input; Vmanual input; Vbase local double; Voffset output; PwrSta input; KTHC_VBlowerdfog_K input; KTHC_VBlowerMin_K input; KTHC_VBlowerMid_K input; KTHC_VBlowerDcCh_K input; KTHC_VBlowerSetLow_K input

== stateflow chart thc/THC/ThermalControl/THCM_Conctrl/CompCtrl/Enabled Subsystem/Chart ==
  state LV1
    en:DTymin=KTHC_DTymin1_K;
  state LV2
    en:DTymin=KTHC_DTymin2_K;
  state LV3
    en:DTymin=KTHC_DTymin3_K;
  state LV4
    en:DTymin=KTHC_DTymin4_K;
  state LV5
    en:DTymin=KTHC_DTymin5_K;
  (default) -> (junction 8)
  (junction 8) -> LV1 [order 1] : [Tamb<KTHC_T1Maxamb_C]
  (junction 8) -> (junction 9) [order 2]
  LV1 -> LV2 : [Tamb>KTHC_T1Maxamb_C]
  LV2 -> LV1 [order 2] : [Tamb<KTHC_T2Minamb_C]
  (junction 9) -> LV2 [order 1] : [Tamb<KTHC_T2Maxamb_C]
  (junction 9) -> (junction 10) [order 2]
  LV2 -> LV3 [order 1] : [Tamb>KTHC_T2Maxamb_C]
  LV3 -> LV2 [order 2] : [Tamb<KTHC_T3Minamb_C]
  (junction 10) -> LV3 [order 1] : [Tamb<KTHC_T3Maxamb_C]
  (junction 10) -> (junction 11) [order 2]
  LV3 -> LV4 [order 1] : [Tamb>KTHC_T3Maxamb_C]
  LV4 -> LV3 [order 2] : [Tamb<KTHC_T4Minamb_C]
  (junction 11) -> LV4 [order 1] : [Tamb<KTHC_T4Maxamb_C]
  (junction 11) -> (junction 12) [order 2]
  LV4 -> LV5 [order 1] : [Tamb>KTHC_T4Maxamb_C]
  LV5 -> LV4 : [Tamb<KTHC_T5Minamb_C]
  (junction 12) -> LV5
  data: Tamb input; KTHC_DTymin1_K input; KTHC_DTymin2_K input; KTHC_DTymin3_K input; KTHC_DTymin4_K input; KTHC_DTymin5_K input; KTHC_T1Maxamb_C input; KTHC_T2Maxamb_C input; KTHC_T3Maxamb_C input; KTHC_T4Maxamb_C input; KTHC_T2Minamb_C input; KTHC_T3Minamb_C input; KTHC_T4Minamb_C input; KTHC_T5Minamb_C input; DTymin output double

== stateflow chart thc/THC/ThermalControl/THCM_Conctrl/APTC/Chart ==
  state APTCPro_FrLe [parallel]
    settings: executionOrder=1
    state Derating
      state State2
        (default) -> (junction 23)
        APTCPro_FrLe.Derating.State2 -> (junction 23) [order 1]
        (junction 23) -> (junction 26) [order 1] : [FD_FrLeAPTCHeatPwr_Cmd>KTHC_DAPTCQ1_W]{FD_FrLeAPTCHeatPwr_Cmd=FD_FrLeAPTCHeatPwr_Cmd-KTHC_DAPTCQ1_W;}
        (junction 23) -> (junction 28) [order 2] : {FD_FrLeAPTCHeatPwr_Cmd=0;}
      state State3
        (default) -> (junction 31)
        APTCPro_FrLe.Derating.State3 -> (junction 31) [order 1]
        (junction 31) -> (junction 32) [order 1] : [FD_FrLeAPTCHeatPwr_Cmd>KTHC_DAPTCQ2_W]{FD_FrLeAPTCHeatPwr_Cmd=FD_FrLeAPTCHeatPwr_Cmd-KTHC_DAPTCQ2_W;}
        (junction 31) -> (junction 33) [order 2] : {FD_FrLeAPTCHeatPwr_Cmd=0;}
      state State4
        (default) -> (junction 39)
        APTCPro_FrLe.Derating.State4 -> (junction 39) [order 1]
        (junction 39) -> (junction 40) [order 1] : [FD_FrLeAPTCHeatPwr_Cmd>KTHC_DAPTCQ3_W]{FD_FrLeAPTCHeatPwr_Cmd=FD_FrLeAPTCHeatPwr_Cmd-KTHC_DAPTCQ3_W;}
        (junction 39) -> (junction 41) [order 2] : {FD_FrLeAPTCHeatPwr_Cmd=0;}
      state State5
      (default) -> APTCPro_FrLe.Derating.State2
      APTCPro_FrLe.Derating.State3 -> APTCPro_FrLe.Derating.State2 [order 1] : [Tventmax_FrLe>KTHC_TventL1_C]
      APTCPro_FrLe.Derating.State2 -> APTCPro_FrLe.Derating.State3 [order 1] : [Tventmax_FrLe<KTHC_TventL2_C]
      APTCPro_FrLe.Derating.State4 -> APTCPro_FrLe.Derating.State3 [order 1] : [Tventmax_FrLe>KTHC_TventL2_C]
      APTCPro_FrLe.Derating.State3 -> APTCPro_FrLe.Derating.State4 [order 2] : [Tventmax_FrLe<KTHC_TventL3_C]
      APTCPro_FrLe.Derating.State5 -> APTCPro_FrLe.Derating.State4 : [Tventmax_FrLe>KTHC_TventL3_C]
      APTCPro_FrLe.Derating.State4 -> APTCPro_FrLe.Derating.State5 [order 2] : [Tventmax_FrLe<KTHC_TventL4_C]
    state PICtrl
      en:FD_FrLeAPTCHeatPwr_Cmd=FD_FrLeAPTC_Cmd;
      du:FD_FrLeAPTCHeatPwr_Cmd=FD_FrLeAPTC_Cmd;
      state Normal
        en:CtrlReset=0;
      state ResetController
        en:CtrlReset=1;
      (default) -> APTCPro_FrLe.PICtrl.Normal
      APTCPro_FrLe.PICtrl.ResetController -> APTCPro_FrLe.PICtrl.Normal
    (default) -> APTCPro_FrLe.PICtrl
    APTCPro_FrLe.PICtrl -> APTCPro_FrLe.Derating : [Tventmax_FrLe>KTHC_TventL1_C]
    APTCPro_FrLe.Derating -> APTCPro_FrLe.PICtrl [order 2] : [FD_FrLeAPTCHeatPwr_Cmd>FD_FrLeAPTC_Cmd]
    APTCPro_FrLe.Derating -> APTCPro_FrLe.PICtrl.ResetController [order 1] : [Tventmax_FrLe<KTHC_TventL5_C]
  state APTCPro_FrRi [parallel]
    settings: executionOrder=2
    state Derating
      state State2
        (default) -> (junction 87)
        APTCPro_FrRi.Derating.State2 -> (junction 87) [order 1]
        (junction 87) -> (junction 88) [order 1] : [FD_FrRiAPTCHeatPwr_Cmd>KTHC_DAPTCQ1_W]{FD_FrRiAPTCHeatPwr_Cmd=FD_FrRiAPTCHeatPwr_Cmd-KTHC_DAPTCQ1_W;}
        (junction 87) -> (junction 89) [order 2] : {FD_FrRiAPTCHeatPwr_Cmd=0;}
      state State3
        (default) -> (junction 58)
        APTCPro_FrRi.Derating.State3 -> (junction 58) [order 1]
        (junction 58) -> (junction 59) [order 1] : [FD_FrRiAPTCHeatPwr_Cmd>KTHC_DAPTCQ2_W]{FD_FrRiAPTCHeatPwr_Cmd=FD_FrRiAPTCHeatPwr_Cmd-KTHC_DAPTCQ2_W;}
        (junction 58) -> (junction 60) [order 2] : {FD_FrRiAPTCHeatPwr_Cmd=0;}
      state State4
        (default) -> (junction 78)
        APTCPro_FrRi.Derating.State4 -> (junction 78) [order 1]
        (junction 78) -> (junction 79) [order 1] : [FD_FrRiAPTCHeatPwr_Cmd>KTHC_DAPTCQ3_W]{FD_FrRiAPTCHeatPwr_Cmd=FD_FrRiAPTCHeatPwr_Cmd-KTHC_DAPTCQ3_W;}
        (junction 78) -> (junction 80) [order 2] : {FD_FrRiAPTCHeatPwr_Cmd=0;}
      state State5
      (default) -> APTCPro_FrRi.Derating.State2
      APTCPro_FrRi.Derating.State3 -> APTCPro_FrRi.Derating.State2 [order 1] : [Tventmax_FrRi>KTHC_TventL1_C]
      APTCPro_FrRi.Derating.State2 -> APTCPro_FrRi.Derating.State3 [order 1] : [Tventmax_FrRi<KTHC_TventL2_C]
      APTCPro_FrRi.Derating.State4 -> APTCPro_FrRi.Derating.State3 [order 1] : [Tventmax_FrRi>KTHC_TventL2_C]
      APTCPro_FrRi.Derating.State3 -> APTCPro_FrRi.Derating.State4 [order 2] : [Tventmax_FrRi<KTHC_TventL3_C]
      APTCPro_FrRi.Derating.State5 -> APTCPro_FrRi.Derating.State4 : [Tventmax_FrRi>KTHC_TventL3_C]
      APTCPro_FrRi.Derating.State4 -> APTCPro_FrRi.Derating.State5 [order 2] : [Tventmax_FrRi<KTHC_TventL4_C]
    state PICtrl
      en:FD_FrRiAPTCHeatPwr_Cmd=FD_FrRiAPTC_Cmd;
      du:FD_FrRiAPTCHeatPwr_Cmd=FD_FrRiAPTC_Cmd;
      state Normal
        en:CtrlReset=0;
      state ResetController
        en:CtrlReset=1;
      (default) -> APTCPro_FrRi.PICtrl.Normal
      APTCPro_FrRi.PICtrl.ResetController -> APTCPro_FrRi.PICtrl.Normal
    (default) -> APTCPro_FrRi.PICtrl
    APTCPro_FrRi.PICtrl -> APTCPro_FrRi.Derating : [Tventmax_FrRi>KTHC_TventL1_C]
    APTCPro_FrRi.Derating -> APTCPro_FrRi.PICtrl [order 2] : [FD_FrRiAPTCHeatPwr_Cmd>FD_FrRiAPTC_Cmd]
    APTCPro_FrRi.Derating -> APTCPro_FrRi.PICtrl.ResetController [order 1] : [Tventmax_FrRi<KTHC_TventL5_C]
  state APTCPro_Rr [parallel]
    settings: executionOrder=3
    state Derating
      state State2
        (default) -> (junction 125)
        APTCPro_Rr.Derating.State2 -> (junction 125) [order 1]
        (junction 125) -> (junction 126) [order 1] : [FD_RrAPTCHeatPwr_Cmd>KTHC_DAPTCQ1_W]{FD_RrAPTCHeatPwr_Cmd=FD_RrAPTCHeatPwr_Cmd-KTHC_DAPTCQ1_W;}
        (junction 125) -> (junction 127) [order 2] : {FD_RrAPTCHeatPwr_Cmd=0;}
      state State3
        (default) -> (junction 96)
        APTCPro_Rr.Derating.State3 -> (junction 96) [order 1]
        (junction 96) -> (junction 97) [order 1] : [FD_RrAPTCHeatPwr_Cmd>KTHC_DAPTCQ2_W]{FD_RrAPTCHeatPwr_Cmd=FD_RrAPTCHeatPwr_Cmd-KTHC_DAPTCQ2_W;}
        (junction 96) -> (junction 98) [order 2] : {FD_RrAPTCHeatPwr_Cmd=0;}
      state State4
        (default) -> (junction 116)
        APTCPro_Rr.Derating.State4 -> (junction 116) [order 1]
        (junction 116) -> (junction 117) [order 1] : [FD_RrAPTCHeatPwr_Cmd>KTHC_DAPTCQ3_W]{FD_RrAPTCHeatPwr_Cmd=FD_RrAPTCHeatPwr_Cmd-KTHC_DAPTCQ3_W;}
        (junction 116) -> (junction 118) [order 2] : {FD_RrAPTCHeatPwr_Cmd=0;}
      state State5
      (default) -> APTCPro_Rr.Derating.State2
      APTCPro_Rr.Derating.State3 -> APTCPro_Rr.Derating.State2 [order 1] : [Tventmax_Rr>KTHC_TventL1_C]
      APTCPro_Rr.Derating.State2 -> APTCPro_Rr.Derating.State3 [order 1] : [Tventmax_Rr<KTHC_TventL2_C]
      APTCPro_Rr.Derating.State4 -> APTCPro_Rr.Derating.State3 [order 1] : [Tventmax_Rr>KTHC_TventL2_C]
      APTCPro_Rr.Derating.State3 -> APTCPro_Rr.Derating.State4 [order 2] : [Tventmax_Rr<KTHC_TventL3_C]
      APTCPro_Rr.Derating.State5 -> APTCPro_Rr.Derating.State4 : [Tventmax_Rr>KTHC_TventL3_C]
      APTCPro_Rr.Derating.State4 -> APTCPro_Rr.Derating.State5 [order 2] : [Tventmax_Rr<KTHC_TventL4_C]
    state PICtrl
      en:FD_RrAPTCHeatPwr_Cmd=FD_RrAPTC_Cmd;
      du:FD_RrAPTCHeatPwr_Cmd=FD_RrAPTC_Cmd;
      state Normal
        en:CtrlReset=0;
      state ResetController
        en:CtrlReset=1;
      (default) -> APTCPro_Rr.PICtrl.Normal
      APTCPro_Rr.PICtrl.ResetController -> APTCPro_Rr.PICtrl.Normal
    (default) -> APTCPro_Rr.PICtrl
    APTCPro_Rr.PICtrl -> APTCPro_Rr.Derating : [Tventmax_Rr>KTHC_TventL1_C]
    APTCPro_Rr.Derating -> APTCPro_Rr.PICtrl [order 2] : [FD_RrAPTCHeatPwr_Cmd>FD_RrAPTC_Cmd]
    APTCPro_Rr.Derating -> APTCPro_Rr.PICtrl.ResetController [order 1] : [Tventmax_Rr<KTHC_TventL5_C]
  data: FD_FrLeAPTC_Cmd input; FD_FrRiAPTC_Cmd input; FD_RrAPTC_Cmd input; Tventmax_FrLe input; Tventmax_FrRi input; Tventmax_Rr input; KTHC_TventL1_C input; KTHC_TventL2_C input; KTHC_TventL3_C input; KTHC_TventL4_C input; KTHC_TventL5_C input; KTHC_DAPTCQ1_W input; KTHC_DAPTCQ2_W input; KTHC_DAPTCQ3_W input; FD_FrLeAPTCHeatPwr_Cmd output double; FD_FrRiAPTCHeatPwr_Cmd output double; FD_RrAPTCHeatPwr_Cmd output double; CtrlReset output boolean

== stateflow chart thc/THC/ThermalControl/THCM_Conctrl/Chart1 ==
  state TambLevel
    state WaitForUpdate
    (default) -> (junction 43)
    WaitForUpdate -> (junction 43) [order 4] : [hasChanged(ECOSW)]
    (junction 43) -> (junction 19)
    WaitForUpdate -> (junction 19) [order 1] : [hasChanged(SetTempZon1St_CMD)]
    (junction 19) -> (junction 25)
    WaitForUpdate -> (junction 25) [order 2] : [hasChanged(SetTempZon2St_CMD)]
    (junction 25) -> (junction 21)
    WaitForUpdate -> (junction 21) [order 3] : [after(KTHC_ECOTambLVT_sec*10,tick)]
    (junction 21) -> (junction 46)
    (junction 46) -> WaitForUpdate [order 1] : [!ECOSW]{alpha=0;beta=0;sigSetTempZon1Stadj=sigSetTempZon1St;sigSetTempZon2Stadj=sigSetTempZon2St;}
    (junction 46) -> (junction 5) [order 2]
    (junction 5) -> (junction 29) [order 1] : [Tamb<KTHC_ECOTambLV1_C]{alpha=KTHC_ECOalpha1_K;beta=KTHC_ECObeta1_K;}
    (junction 5) -> (junction 7) [order 2]
    (junction 29) -> (junction 31)
    (junction 7) -> (junction 31) [order 1] : [Tamb<KTHC_ECOTambLV2_C]{alpha=KTHC_ECOalpha2_K;beta=KTHC_ECObeta2_K;}
    (junction 7) -> (junction 10) [order 2]
    (junction 31) -> (junction 34)
    (junction 10) -> (junction 34) [order 1] : [Tamb<KTHC_ECOTambLV3_C]{alpha=KTHC_ECOalpha3_K;beta=KTHC_ECObeta3_K;}
    (junction 10) -> (junction 13) [order 2]
    (junction 34) -> (junction 37)
    (junction 13) -> (junction 37) [order 1] : [Tamb<KTHC_ECOTambLV4_C]{alpha=KTHC_ECOalpha4_K;beta=KTHC_ECObeta4_K;}
    (junction 13) -> (junction 16) [order 2]
    (junction 37) -> (junction 40)
    (junction 16) -> (junction 40) [order 1] : [Tamb<KTHC_ECOTambLV5_C]{alpha=KTHC_ECOalpha5_K;beta=KTHC_ECObeta5_K;}
    (junction 16) -> (junction 110) [order 2]
    (junction 40) -> (junction 97)
    (junction 110) -> (junction 97) [order 1] : [Tamb<KTHC_ECOTambLV6_C]{alpha=KTHC_ECOalpha6_K;beta=KTHC_ECObeta6_K;}
    (junction 110) -> (junction 107) [order 2]
    (junction 97) -> (junction 95)
    (junction 107) -> (junction 95) [order 1] : [Tamb<KTHC_ECOTambLV7_C]{alpha=KTHC_ECOalpha7_K;beta=KTHC_ECObeta7_K;}
    (junction 107) -> (junction 103) [order 2]
    (junction 95) -> (junction 100)
    (junction 103) -> (junction 100) [order 1] : [Tamb<KTHC_ECOTambLV8_C]{alpha=KTHC_ECOalpha8_K;beta=KTHC_ECObeta8_K;}
    (junction 103) -> (junction 94) [order 2]
    (junction 100) -> (junction 102)
    (junction 94) -> (junction 102) : {alpha=KTHC_ECOalpha9_K;beta=KTHC_ECObeta9_K;}
    (junction 102) -> (junction 54) [order 1] : [sigSetTempZon1St<Tamb]
        | {sigSetTempZon1Stadj=sigSetTempZon1St-(sigSetTempZon1St-Tamb)*alpha;}
    (junction 102) -> (junction 55) [order 2]
    (junction 54) -> (junction 57)
    (junction 55) -> (junction 57) : {sigSetTempZon1Stadj=sigSetTempZon1St-(sigSetTempZon1St-Tamb)*beta;}
    (junction 57) -> WaitForUpdate [order 1] : [sigSetTempZon2St<Tamb]
        | {sigSetTempZon2Stadj=sigSetTempZon2St-(sigSetTempZon2St-Tamb)*alpha;}
    (junction 57) -> (junction 62) [order 2]
    (junction 62) -> WaitForUpdate : {sigSetTempZon2Stadj=sigSetTempZon2St-(sigSetTempZon2St-Tamb)*beta;}
  data: KTHC_ECOTambLV1_C input; KTHC_ECOTambLV2_C input; KTHC_ECOTambLV3_C input; KTHC_ECOTambLV4_C input; KTHC_ECOTambLV5_C input; KTHC_ECOTambLV6_C input; KTHC_ECOTambLV7_C input; KTHC_ECOTambLV8_C input; KTHC_ECOTambLVT_sec input; KTHC_ECOalpha1_K input; KTHC_ECOalpha2_K input; KTHC_ECOalpha3_K input; KTHC_ECOalpha4_K input; KTHC_ECOalpha5_K input; KTHC_ECOalpha6_K input; KTHC_ECOalpha7_K input; KTHC_ECOalpha8_K input; KTHC_ECObeta1_K input; KTHC_ECObeta2_K input; KTHC_ECObeta3_K input; KTHC_ECObeta4_K input; KTHC_ECObeta5_K input; KTHC_ECOalpha9_K input; KTHC_ECObeta6_K input; KTHC_ECObeta7_K input; KTHC_ECObeta8_K input; KTHC_ECObeta9_K input; Tamb input; sigSetTempZon1St input; SetTempZon1St_CMD input; sigSetTempZon1Stadj output double; alpha local double; beta local double; sigSetTempZon2St input; SetTempZon2St_CMD input; sigSetTempZon2Stadj output double; ECOSW input

== stateflow chart thc/THC/ThermalControl/THCM_Conctrl/CompCtrl/Enabled Subsystem1/Chart ==
  state Level1
    en:Bat_In_TempSetPoint=KTHC_T1winSetpointBC_C;
  state Level2
    en:Bat_In_TempSetPoint=KTHC_T2winSetpointBC_C;
  state Level3
    en:Bat_In_TempSetPoint=KTHC_T3winSetpointBC_C;
  state Level4
    en:Bat_In_TempSetPoint=KTHC_T4winSetpointBC_C;
  state Level5
    en:Bat_In_TempSetPoint=KTHC_T5winSetpointBC_C;
  (default) -> Level1
  Level1 -> Level2 : [TBMax>KTHC_T1MaxBC_C]
  Level2 -> Level1 [order 2] : [TBMax<KTHC_T2MinBC_C]
  Level2 -> Level3 [order 1] : [TBMax>KTHC_T2MaxBC_C]
  Level3 -> Level2 [order 2] : [TBMax<KTHC_T3MinBC_C]
  Level3 -> Level4 [order 1] : [TBMax>KTHC_T3MaxBC_C]
  Level4 -> Level3 [order 1] : [TBMax<KTHC_T4MinBC_C]
  Level4 -> Level5 [order 2] : [TBMax>KTHC_T4MaxBC_C]
  Level5 -> Level4 : [TBMax<KTHC_T5MinBC_C]
  data: TBMax input; Bat_In_TempSetPoint output; KTHC_T1MaxBC_C input; KTHC_T2MinBC_C input; KTHC_T2MaxBC_C input; KTHC_T3MinBC_C input; KTHC_T3MaxBC_C input; KTHC_T4MinBC_C input; KTHC_T4MaxBC_C input; KTHC_T5MinBC_C input; KTHC_T1winSetpointBC_C input; KTHC_T2winSetpointBC_C input; KTHC_T3winSetpointBC_C input; KTHC_T4winSetpointBC_C input; KTHC_T5winSetpointBC_C input

== stateflow chart thc/THC/ThermalControl/THCM_Conctrl/APTC/Chart1 ==
  state OFF
    en:APTCset=0;
  state ONOFF
    state ON
      en:APTCset=KTHC_APTCQminC_W;
    state OFF
      en:APTCset=0;
    (default) -> ON
    ON -> ONOFF.OFF : [after(KTHC_APTCQonT_cnt,tick)]
    ONOFF.OFF -> ON : [after(KTHC_APTCQoffT_cnt,tick)]
  (default) -> OFF
  OFF -> ONOFF : [APTCPID==8]
  ONOFF -> OFF : [APTCPID!=8]
  data: KTHC_APTCQminC_W input; APTCPID input; KTHC_APTCQonT_cnt input; KTHC_APTCQoffT_cnt input; APTCset output double
